simulink model "P4simulink"  (R2022b)
settings: Solver=VariableStepAuto  StartTime=0.0  StopTime=10.0  RelTol=1e-3
values from neighbouring files (symbols this model uses):
  K1 = -1    [P4.m]
  K2 = 0.8    [P4.m]
  Treshold_y = 10    [P4.m]
  V = 15    [P4.m]
  Vy_Inicial = 1    [P4.m]
libraries: simulink x2
settings Model: Creator=TERESA NOGUEIRA  LastModifiedBy=TERESA NOGUEIRA
settings SolverCC: ZeroCrossAlgorithm=Adaptive

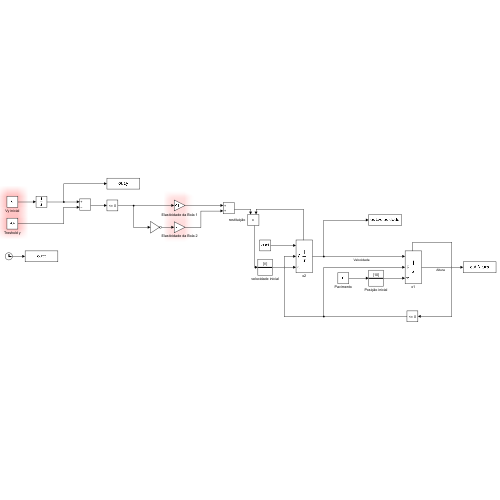
[thumbnail: Simulink's stored preview of the top-level diagram]
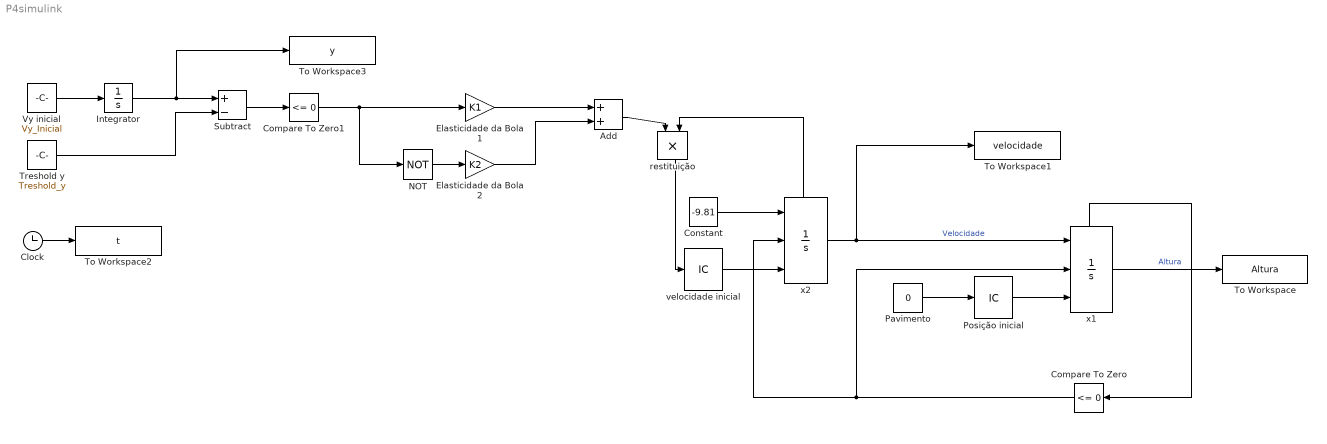
== system P4simulink ==
  Add : Sum
  Clock : Clock
      settings: Decimation=200
  Compare To Zero : simulink/Logic and Bit Operations/Compare To Zero  relop=<=  OutDataTypeStr=boolean
  Compare To Zero1 : simulink/Logic and Bit Operations/Compare To Zero  relop=<=  OutDataTypeStr=boolean
  Constant : Constant  Value=-9.81
  Elasticidade da Bola 1 : Gain  Gain=K1
  Elasticidade da Bola 2 : Gain  Gain=K2
  Integrator : Integrator  ContinuousStateAttributes='xpos'
  NOT : Logic  Operator=NOT  IconShape=distinctive  AllPortsSameDT=off  OutDataTypeStr=boolean
  Pavimento : Constant  Value=0
  Posição inicial : InitialCondition  Value=10
  Subtract : Sum  Inputs=+-
  To Workspace : ToWorkspace  VariableName=Altura  SampleTime=-1
      settings: Save2DSignal=2-D array (concatenate along first dimension)
  To Workspace1 : ToWorkspace  VariableName=velocidade  SampleTime=-1
      settings: Save2DSignal=2-D array (concatenate along first dimension)
  To Workspace2 : ToWorkspace  VariableName=t  SampleTime=-1
      settings: Save2DSignal=2-D array (concatenate along first dimension)
  To Workspace3 : ToWorkspace  VariableName=y  SampleTime=-1
  Treshold y : Constant  Value=Treshold_y
  Vy inicial : Constant  Value=Vy_Inicial
  restituição : Product
  velocidade inicial : InitialCondition  Value=V
  x1 : Integrator  ExternalReset=rising  InitialConditionSource=external  ShowStatePort=on
  x2 : Integrator  ExternalReset=rising  InitialConditionSource=external  ShowStatePort=on
  wires:
  Treshold y/1 -> Subtract/2
  x2/State -> restituição/2
  Vy inicial/1 -> Integrator/1
  Pavimento/1 -> Posição inicial/1
  x1/State -> Compare To Zero/1
  x1/1 -> To Workspace/1  "Altura"
  Clock/1 -> To Workspace2/1
  Constant/1 -> x2/1
  Posição inicial/1 -> x1/3
  velocidade inicial/1 -> x2/3
  Integrator/1 -> Subtract/1, To Workspace3/1
  x2/1 -> To Workspace1/1, x1/1  "Velocidade"
  Compare To Zero1/1 -> NOT/1, Elasticidade da Bola 1/1
  NOT/1 -> Elasticidade da Bola 2/1
  Subtract/1 -> Compare To Zero1/1
  Elasticidade da Bola 1/1 -> Add/1
  Compare To Zero/1 -> x2/2, x1/2
  Elasticidade da Bola 2/1 -> Add/2
  restituição/1 -> velocidade inicial/1
  Add/1 -> restituição/1
